simulink model "projectSNS"  (R2023b)
settings: Solver=VariableStepAuto  StartTime=0.0  StopTime=10.0  RelTol=1e-3
libraries: dspfdesign x5, simulink x5, dspvision x2, dspsnks4 x1
settings Model: Creator=HP  LastModifiedBy=PMYLS
settings ModelReferenceCC: EnableRefExpFcnMdlSchedulingChecks=on
settings RTWCC: GenCodeOnly=on  GenerateReport=on  LaunchReport=on

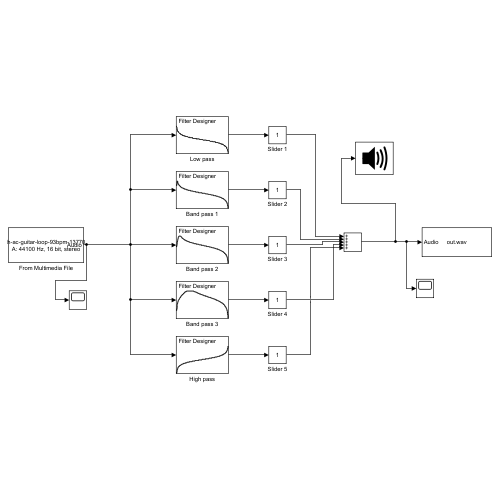
[thumbnail: Simulink's stored preview of the top-level diagram]
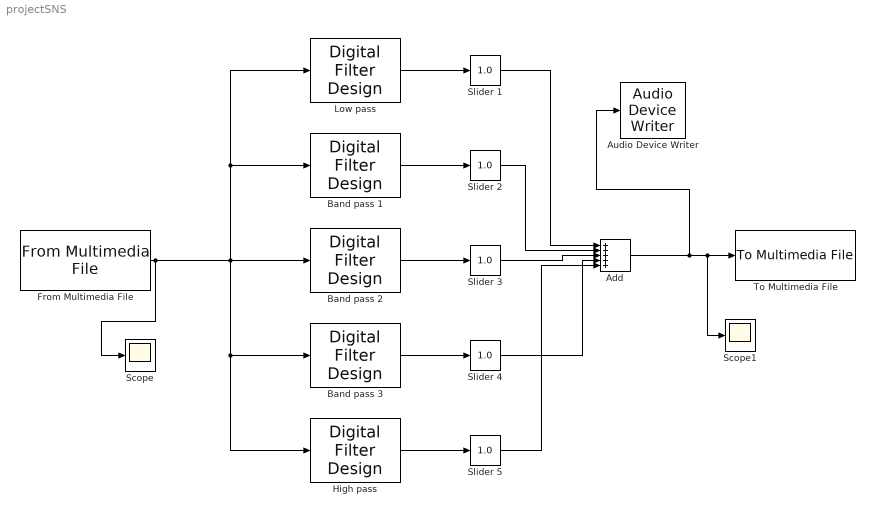
== system projectSNS ==
  Add : Sum  Inputs=+++++
  Audio Device Writer : dspsnks4/Audio Device Writer  Driver=DirectSound  Device=Default  InheritSampleRate=on  SampleRate=44100  BitDepth=16-bit integer  BufferSize=4096  NumBuffers=10  DefaultOutputChannelMapping=on  OutputChannelMapping=1:2  OutputNumUnderrunSamples=off  DriverIdx=1  DeviceWarnFlag=''
  Band pass 1 : dspfdesign/Digital Filter Design  mwdsp_browser_bugfix_var=off
  Band pass 2 : dspfdesign/Digital Filter Design  mwdsp_browser_bugfix_var=off
  Band pass 3 : dspfdesign/Digital Filter Design  mwdsp_browser_bugfix_var=off
  From Multimedia File : dspvision/From Multimedia File  inputFilename=C:\Users\PMLS\Documents\MATLAB\Examples\R2023b\simulink_general\sldemo_zeroxingExample\proj\smooth-ac-guitar-loop-93bpm-137706.wav  readRange=[1 Inf]  loop=on  numPlays=inf  outputStreams=Audio only  videoDataType=single  audioDataType=double  inheritSampleTime=on  userDefinedSampleTime=1/30  noAudioOutput=off  isIntensityVideo=off  fourcc=RGB  colorVideoFormat=Separate color signals  outputEOF=off  dataOrg=Column-major  audioFrameSize=1024  computeAudioFrameSize=off  outSamplingMode=Sample based
  High pass : dspfdesign/Digital Filter Design  mwdsp_browser_bugfix_var=off
  Low pass : dspfdesign/Digital Filter Design  mwdsp_browser_bugfix_var=off
  Scope : Scope
  Scope1 : Scope
  Slider {1..5} (5 alike) : simulink/Math Operations/Slider Gain  gain=1.0  low=0  high=10
  To Multimedia File : dspvision/To Multimedia File  outputFilename=out.wav  streamSelection=Audio only  videoCompressor=None (uncompressed)  audioCompressor=None (uncompressed)  imagePorts=Separate color signals  fileType=WAV  audioDatatype=16-bit integer  fourcc=RGB  videoQuality=75  mj2000CompFactor=10
  wires:
  High pass/1 -> Slider 5/1
  Band pass 3/1 -> Slider 4/1
  Band pass 2/1 -> Slider 3/1
  Band pass 1/1 -> Slider 2/1
  Low pass/1 -> Slider 1/1
  Slider 1/1 -> Add/1
  Slider 2/1 -> Add/2
  Slider 3/1 -> Add/3
  Slider 4/1 -> Add/4
  Slider 5/1 -> Add/5
  From Multimedia File/1 -> Scope/1, High pass/1, Band pass 3/1, Band pass 1/1, Low pass/1, Band pass 2/1
  Add/1 -> Audio Device Writer/1, Scope1/1, To Multimedia File/1
